simulink model "MatlabTestSerial3"  (R2018b)
settings: Solver=ode3  StartTime=0.0  StopTime=20.0  FixedStep=0.5  RelTol=1e-3
undefined symbols (not defined in the file or in its folder): fclose, s1
libraries: realtime_pacer_lib x1
settings Model: Creator=marci  LastModifiedBy=marci

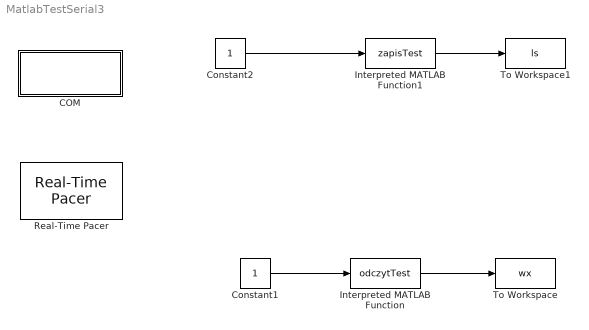
== system MatlabTestSerial3 ==
  COM : Subsystem  StartFcn=|  StopFcn=fclose(s1);
      | global s1;
      | if ~isempty(instrfind)
      |      fclose(instrfind);
      |       delete(instrfind);
      |  end
      | s1 = serial("COM4","BaudRate",115200);
      | 
      | fopen(s1);
  Constant1 : Constant  SampleTime=0.5
  Constant2 : Constant  SampleTime=0.5
  Interpreted MATLAB Function : MATLABFcn  MATLABFcn=odczytTest  OutputDimensions=2  Output1D=off
  Interpreted MATLAB Function1 : MATLABFcn  MATLABFcn=zapisTest
  Real-Time Pacer : realtime_pacer_lib/Real-Time Pacer  simTimePerRealTime=1
  To Workspace : ToWorkspace  VariableName=wx  SampleTime=-1
  To Workspace1 : ToWorkspace  VariableName=ls  SampleTime=-1
  wires:
  Interpreted MATLAB Function/1 -> To Workspace/1
  Constant1/1 -> Interpreted MATLAB Function/1
  Interpreted MATLAB Function1/1 -> To Workspace1/1
  Constant2/1 -> Interpreted MATLAB Function1/1

== system MatlabTestSerial3/COM ==
